simulink model "Lab3BLine"  (R2020a)
settings: Solver=VariableStepAuto  StartTime=0.0  StopTime=10.0  RelTol=1e-3
values from neighbouring files (symbols this model uses):
  K = place(Ad,Bd,pz)    [Lab3B.m]    (also in PenUpTest.m)
  Lo = place(Ad',Cd',pL)'    [Lab3B.m]    (also in PenUpTest.m)
  T = 0.005    [Lab3B.m]    (also in PenUpTest.m)
  X0 = [0;0;5*pi/180;0]    [Lab3B.m]    (also in PenUpTest.m = [0;0;pi/4;0])
  X_obs_0 = [0;0;0;0]    [Lab3B.m]    (also in PenUpTest.m)
undefined symbols (not defined in the file or in its folder): Ad, Bd, Cd
libraries: dspsrcs4 x1
settings Model: Creator=andre  LastModifiedBy=andre

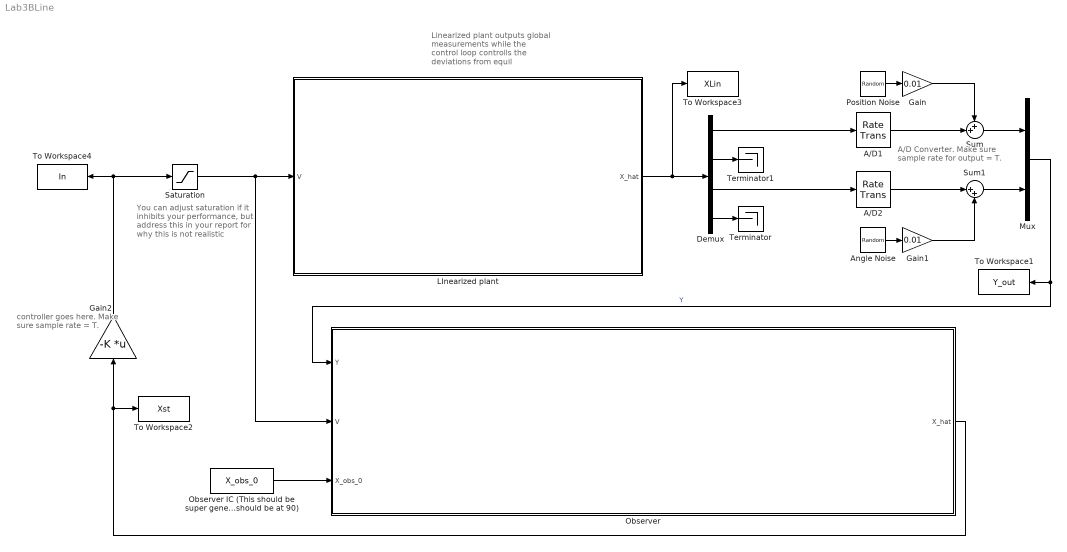
== system Lab3BLine ==
  note: You can adjust saturation if it inhibits your performance, but address this in your report for why this is not realistic
  note: controller goes here.
      | Make sure sample
      | rate = T.
  note: A/D Converter.
      | Make sure sample rate for output = T.
  note: Linearized plant outputs global measurements while the control loop controlls the deviations from equil
  A/D1 : RateTransition  OutPortSampleTime=T
  A/D2 : RateTransition  OutPortSampleTime=T
  "Angle Noise " : RandomNumber  Variance=0.5  SampleTime=T
  Demux : Demux
  Gain : Gain  Gain=0.01
  Gain1 : Gain  Gain=0.01
  Gain2 : Gain  Gain=-K  Multiplication=Matrix(K*u) (u vector)
  LInearized plant : Subsystem
  Mux : Mux  Inputs=2
  Observer : Subsystem
  "Observer IC (This should be super generic - for example, if plant starts at 80 degrees, then this should be at 90)" : Constant  Value=X_obs_0
  Position Noise : RandomNumber  Variance=0.5  SampleTime=T
  Saturation : Saturate  UpperLimit=20  LowerLimit=-20
  Sum : Sum  Inputs=++|
  Sum1 : Sum  Inputs=|++
  Terminator : Terminator
  Terminator1 : Terminator
  To Workspace1 : ToWorkspace  VariableName=Y_out  SampleTime=-1
  To Workspace2 : ToWorkspace  VariableName=Xst  SampleTime=-1
  To Workspace3 : ToWorkspace  VariableName=XLin  SampleTime=-1
  To Workspace4 : ToWorkspace  VariableName=In  SampleTime=-1
  wires:
  Gain1/1 -> Sum1/2
  Position Noise/1 -> Gain/1
  "Observer IC (This should be super generic - for example, if plant starts at 80 degrees, then this should be at 90)"/1 -> Observer/3(X_obs_0)
  A/D2/1 -> Sum1/1
  Demux/1 -> A/D1/1
  Observer/1("X_hat ") -> To Workspace2/1, Gain2/1
  A/D1/1 -> Sum/2
  Gain2/1 -> Saturation/1, To Workspace4/1
  Gain/1 -> Sum/1
  Sum/1 -> Mux/1
  Sum1/1 -> Mux/2
  Mux/1 -> Observer/1(Y), To Workspace1/1  "Y"
  "Angle Noise "/1 -> Gain1/1
  LInearized plant/1("X_hat ") -> To Workspace3/1, Demux/1
  Saturation/1 -> Observer/2(V), LInearized plant/1(V)
  Demux/3 -> A/D2/1
  Demux/2 -> Terminator1/1
  Demux/4 -> Terminator/1

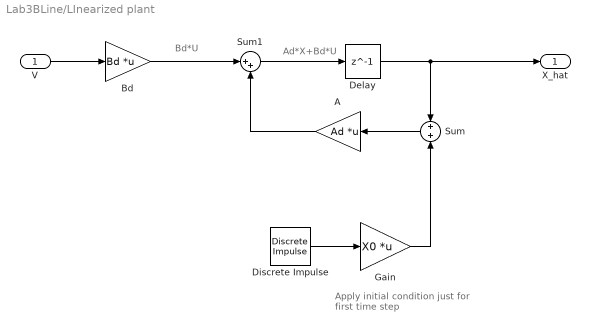
== system Lab3BLine/LInearized plant ==
  note: Bd*U
  note: Ad*X+Bd*U
  note: Apply initial condition
      | just for first time step
  V : Inport
  A : Gain  Gain=Ad  Multiplication=Matrix(K*u) (u vector)
  Bd : Gain  Gain=Bd  Multiplication=Matrix(K*u) (u vector)
  Delay : Delay  DelayLength=1
  Discrete Impulse : dspsrcs4/Discrete  Impulse  Delay=0  SampleTime=T  FrameSample=1  OutputFrames=off  dataType=double  isSigned=on  wordLen=16  udDataType=sfix(16)  fracBitsMode=Best precision  numFracBits=15  OutDataTypeStr=double  LastOutDataTypeStr=double
  Gain : Gain  Gain=X0  Multiplication=Matrix(K*u) (u vector)
  Sum : Sum  Inputs=+|+
  Sum1 : Sum  Inputs=|++
  "X_hat " : Outport  VectorParamsAs1DForOutWhenUnconnected=off
  wires:
  V/1 -> Bd/1
  Bd/1 -> Sum1/1
  A/1 -> Sum1/2
  Sum1/1 -> Delay/1
  Delay/1 -> Sum/1, "X_hat "/1
  Sum/1 -> A/1
  Gain/1 -> Sum/2
  Discrete Impulse/1 -> Gain/1

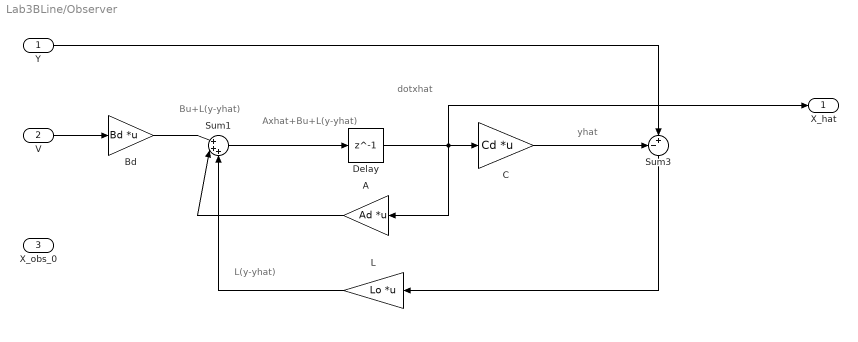
== system Lab3BLine/Observer ==
  note: L(y-yhat)
  note: Bu+L(y-yhat)
  note: Axhat+Bu+L(y-yhat)
  note: dotxhat
  note: yhat
  Y : Inport
  V : Inport  Port=2
  X_obs_0 : Inport  Port=3
  A : Gain  Gain=Ad  Multiplication=Matrix(K*u) (u vector)
  Bd : Gain  Gain=Bd  Multiplication=Matrix(K*u) (u vector)
  C : Gain  Gain=Cd  Multiplication=Matrix(K*u) (u vector)
  Delay : Delay  DelayLength=1
  L : Gain  Gain=Lo  Multiplication=Matrix(K*u) (u vector)
  Sum1 : Sum  Inputs=|+++
  Sum3 : Sum  Inputs=-+|
  "X_hat " : Outport  VectorParamsAs1DForOutWhenUnconnected=off
  wires:
  V/1 -> Bd/1
  L/1 -> Sum1/3
  Bd/1 -> Sum1/1
  A/1 -> Sum1/2
  Sum1/1 -> Delay/1
  C/1 -> Sum3/1
  Sum3/1 -> L/1
  Delay/1 -> A/1, C/1, "X_hat "/1
  Y/1 -> Sum3/2
